simulink model "Simulator_PMU_v4_ons"  (Simulink 8.3)
settings: Solver=FixedStepDiscrete  StartTime=0.0  StopTime=5  FixedStep=1/(60*32)  RelTol=1e-3
undefined symbols (not defined in the file or in its folder): j
libraries: dspbuff3 x5, dspsigops x3, dspxfrm3 x3, simulink x3
settings Model: Creator=dotta  LastModifiedBy=dotta  BufferReuse=off
settings OptimizationCC: BlockReduction=off  InlineParams=on  BufferReuse=off  ExpressionDepthLimit=2147483647
settings DebuggingCC: SigSpecEnsureSampleTimeMsg=none  FcnCallInpInsideContextMsg=UseLocalSettings  StrictBusMsg=Warning
settings SFSimCC: SimParseCustomCode=off

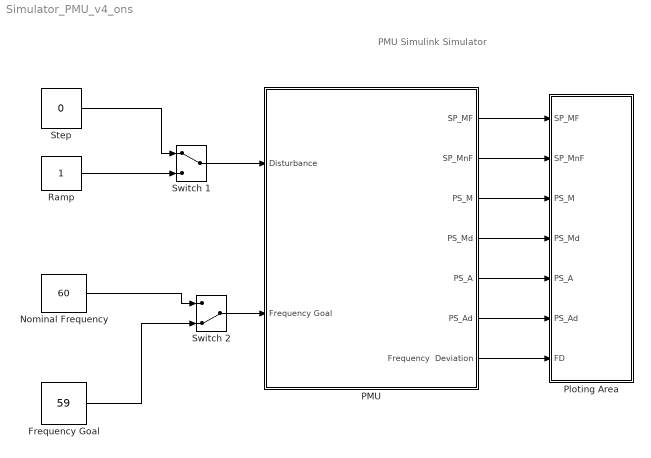
== system Simulator_PMU_v4_ons ==
  note: PMU Simulink Simulator
  Frequency Goal : Constant  Value=59
  Nominal Frequency : Constant  Value=60
  PMU : Subsystem
  Ploting Area : Subsystem
  Ramp : Constant
  Step : Constant  Value=0
  "Switch 1 " : ManualSwitch
  "Switch 2 " : ManualSwitch  CurrentSetting=0
  wires:
  PMU/1(SP_MF) -> Ploting Area/1(SP_MF)
  PMU/2(SP_MnF) -> Ploting Area/2(SP_MnF)
  PMU/4(PS_Md) -> Ploting Area/4(PS_Md)
  PMU/6(PS_Ad) -> Ploting Area/6(PS_Ad)
  Step/1 -> "Switch 1 "/1
  Ramp/1 -> "Switch 1 "/2
  "Switch 2 "/1 -> PMU/2(Frequency Goal)
  PMU/3(PS_M) -> Ploting Area/3(PS_M)
  PMU/5(PS_A) -> Ploting Area/5(PS_A)
  PMU/7(Frequency  Deviation) -> Ploting Area/7(FD)
  Nominal Frequency/1 -> "Switch 2 "/1
  Frequency Goal/1 -> "Switch 2 "/2
  "Switch 1 "/1 -> PMU/1(Disturbance)

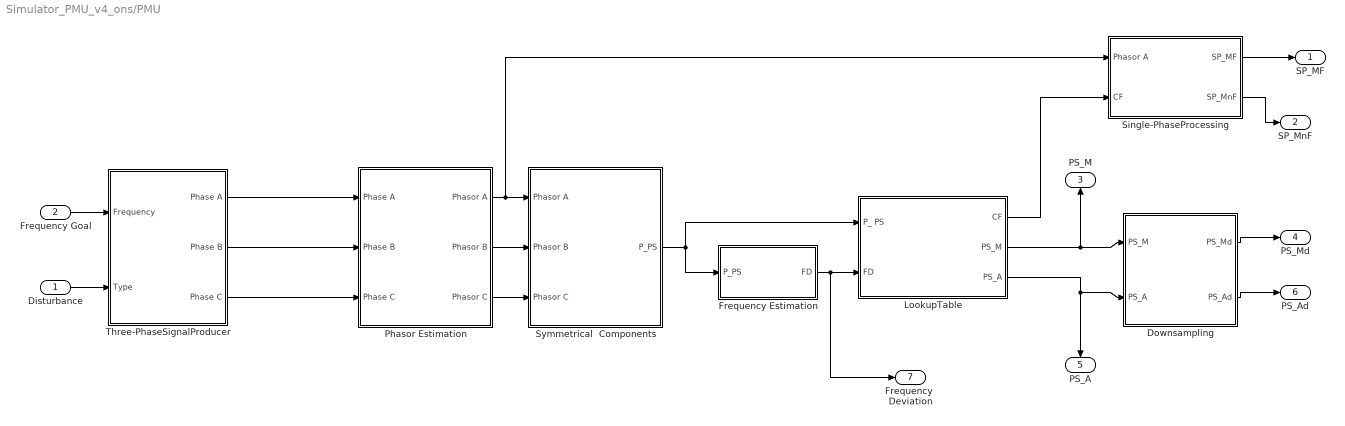
== system Simulator_PMU_v4_ons/PMU ==
  Disturbance : Inport
  Frequency Goal : Inport  Port=2
  Downsampling : Subsystem
  Frequency Estimation : Subsystem
  LookupTable : Subsystem
  Phasor Estimation : Subsystem
  Single-PhaseProcessing : Subsystem
  Symmetrical  Components : Subsystem
  Three-PhaseSignalProducer : Subsystem
  SP_MF : Outport
  SP_MnF : Outport  Port=2
  PS_M : Outport  Port=3
  PS_Md : Outport  Port=4
  PS_A : Outport  Port=5
  PS_Ad : Outport  Port=6
  Frequency  Deviation : Outport  Port=7
  wires:
  Phasor Estimation/1(Phasor A) -> Single-PhaseProcessing/1(Phasor A), Symmetrical  Components/1(Phasor A)
  Symmetrical  Components/1(P_PS) -> Frequency Estimation/1(P_PS), LookupTable/1(P_ PS)
  LookupTable/2(PS_M) -> Downsampling/1(PS_M), PS_M/1
  LookupTable/3(PS_A) -> Downsampling/2(PS_A), PS_A/1
  Frequency Estimation/1(FD) -> LookupTable/2(FD), Frequency  Deviation/1
  LookupTable/1(CF) -> Single-PhaseProcessing/2(CF)
  Phasor Estimation/2(Phasor B) -> Symmetrical  Components/2(Phasor B)
  Phasor Estimation/3(Phasor C) -> Symmetrical  Components/3(Phasor C)
  Single-PhaseProcessing/1(SP_MF) -> SP_MF/1
  Single-PhaseProcessing/2(SP_MnF) -> SP_MnF/1
  Downsampling/1(" PS_Md") -> PS_Md/1
  Frequency Goal/1 -> Three-PhaseSignalProducer/1(Frequency)
  Downsampling/2(PS_Ad) -> PS_Ad/1
  Disturbance/1 -> Three-PhaseSignalProducer/2(Type)
  Three-PhaseSignalProducer/1(Phase A) -> Phasor Estimation/1(" Phase A")
  Three-PhaseSignalProducer/2(Phase B) -> Phasor Estimation/2(Phase B)
  Three-PhaseSignalProducer/3(Phase C) -> Phasor Estimation/3(Phase C)

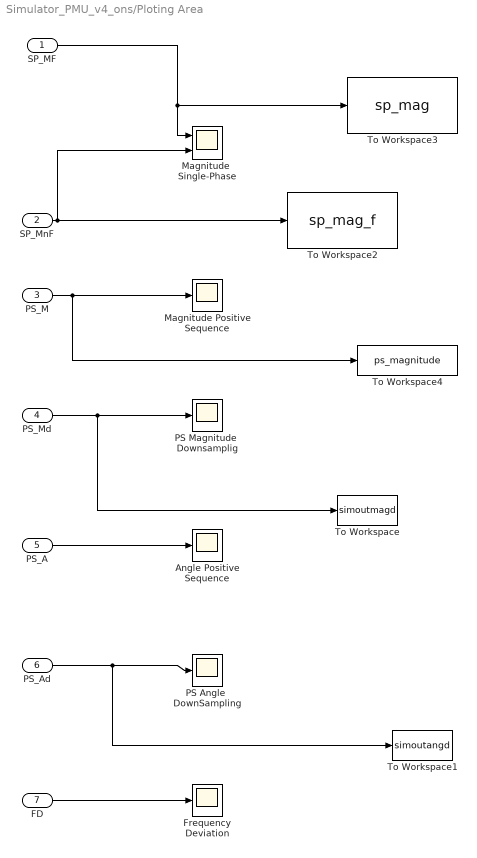
== system Simulator_PMU_v4_ons/Ploting Area ==
  SP_MF : Inport
  SP_MnF : Inport  Port=2
  PS_M : Inport  Port=3
  PS_Md : Inport  Port=4
  PS_A : Inport  Port=5
  PS_Ad : Inport  Port=6
  FD : Inport  Port=7
  Angle Positive Sequence : Scope
      settings: YMin=-3.5  YMax=3.5  SaveName=ScopeData2  MaxDataPoints=10000
  Frequency Deviation : Scope
      settings: YMin=13.85  YMax=15  SaveName=ScopeData3  MaxDataPoints=10000
  Magnitude  Single-Phase : Scope  NumInputPorts=2
      settings: YMin=0.999~0.991  YMax=1.001~1.009  SaveName=ScopeData5  MaxDataPoints=10000
  Magnitude Positive Sequence : Scope
      settings: YMin=0.9993  YMax=1.00025  MaxDataPoints=10000
  PS Angle  DownSampling : Scope
      settings: YMin=-175  YMax=200  SaveName=ScopeData6  MaxDataPoints=10000
  PS Magnitude  Downsamplig : Scope
      settings: YMin=0.95  YMax=1.05  MaxDataPoints=10000
  To Workspace : ToWorkspace  VariableName=simoutmagd  SaveFormat=Structure With Time  SampleTime=-1
  To Workspace1 : ToWorkspace  VariableName=simoutangd  SaveFormat=Structure With Time  SampleTime=-1
  To Workspace2 : ToWorkspace  VariableName=sp_mag_f  SaveFormat=Structure  SampleTime=-1
  To Workspace3 : ToWorkspace  VariableName=sp_mag  SaveFormat=Structure  SampleTime=-1
  To Workspace4 : ToWorkspace  VariableName=ps_magnitude  SaveFormat=Structure With Time  SampleTime=-1
  wires:
  SP_MF/1 -> Magnitude  Single-Phase/1, To Workspace3/1
  SP_MnF/1 -> Magnitude  Single-Phase/2, To Workspace2/1
  PS_M/1 -> Magnitude Positive Sequence/1, To Workspace4/1
  PS_Md/1 -> PS Magnitude  Downsamplig/1, To Workspace/1
  PS_A/1 -> Angle Positive Sequence/1
  PS_Ad/1 -> PS Angle  DownSampling/1, To Workspace1/1
  FD/1 -> Frequency Deviation/1

== system Simulator_PMU_v4_ons/PMU/Downsampling ==
  PS_M : Inport
  PS_A : Inport  Port=2
  Downsample A : dspsigops/Downsample  N=32  phase=0  InputProcessing=Inherited (this choice will be removed - see release notes)  RateOptions=Enforce single-rate processing  smode=Allow multirate  fmode=Maintain input frame size  ic=0
  Downsample M : dspsigops/Downsample  N=32  phase=0  InputProcessing=Inherited (this choice will be removed - see release notes)  RateOptions=Enforce single-rate processing  smode=Allow multirate  fmode=Maintain input frame size  ic=0
  Gain : Gain  Gain=180/pi
  " PS_Md" : Outport
  PS_Ad : Outport  Port=2
  wires:
  Downsample M/1 -> " PS_Md"/1
  PS_M/1 -> Downsample M/1
  PS_A/1 -> Downsample A/1
  Gain/1 -> PS_Ad/1
  Downsample A/1 -> Gain/1

== system Simulator_PMU_v4_ons/PMU/Frequency Estimation ==
  P_PS : Inport
  Complex to Magnitude-Angle : ComplexToMagnitudeAngle  Output=Angle
  Frequency Buffer : dspbuff3/Buffer  N=32*2+1  V=32*2-1  ic=0
  Frequency Datalog : ToWorkspace  VariableName=simoutf  SampleTime=-1
  Frequency  Estimation : MATLABFcn  MATLABFcn=freq_angle  Output1D=off
  FD : Outport
  wires:
  Frequency Buffer/1 -> Frequency  Estimation/1
  Frequency  Estimation/1 -> Frequency Datalog/1, FD/1
  Complex to Magnitude-Angle/1 -> Frequency Buffer/1
  P_PS/1 -> Complex to Magnitude-Angle/1

== system Simulator_PMU_v4_ons/PMU/LookupTable ==
  P_ PS : Inport
  FD : Inport  Port=2
  Complex to Magnitude-Angle : ComplexToMagnitudeAngle
  Divide : Product  Inputs=*/
  P_n Estimation : Subsystem
  Reshape : Reshape
  CF : Outport
  PS_M : Outport  Port=2
  PS_A : Outport  Port=3
  wires:
  Divide/1 -> Complex to Magnitude-Angle/1
  FD/1 -> Reshape/1
  Complex to Magnitude-Angle/1 -> PS_M/1
  Complex to Magnitude-Angle/2 -> PS_A/1
  P_ PS/1 -> Divide/1
  P_n Estimation/1(P_n) -> Divide/2, CF/1
  Reshape/1 -> P_n Estimation/1(Frequency Deviation)

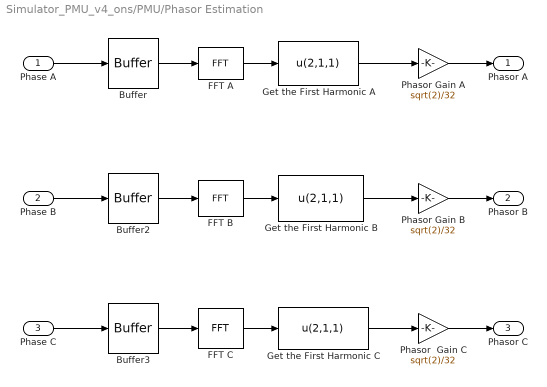
== system Simulator_PMU_v4_ons/PMU/Phasor Estimation ==
  " Phase A" : Inport
  Phase B : Inport  Port=2
  Phase C : Inport  Port=3
  Buffer : dspbuff3/Buffer  N=32  V=31  ic=0
  Buffer2 : dspbuff3/Buffer  N=32  V=31  ic=0
  Buffer3 : dspbuff3/Buffer  N=32  V=31  ic=0
  FFT A : dspxfrm3/FFT  CompMethod=Table lookup  TableOpt=HYBRID  TableOptActive=Speed  BitRevOrder=off  InheritFFTLength=on  FFTLength=31  SkipNorm=off  firstCoeffDataTypeStr=Inherit: Same word length as input  firstCoeffLastDataTypeStr=Inherit: Same word length as input  outputMin=[]  outputMax=[]  roundingMode=Round  overflowMode=off
  FFT B : dspxfrm3/FFT  CompMethod=Table lookup  TableOpt=HYBRID  TableOptActive=Speed  BitRevOrder=off  InheritFFTLength=on  FFTLength=32  SkipNorm=off  firstCoeffDataTypeStr=Inherit: Same word length as input  firstCoeffLastDataTypeStr=Inherit: Same word length as input  outputMin=[]  outputMax=[]  roundingMode=Round  overflowMode=off
  FFT C : dspxfrm3/FFT  CompMethod=Table lookup  TableOpt=HYBRID  TableOptActive=Speed  BitRevOrder=off  InheritFFTLength=on  FFTLength=32  SkipNorm=off  firstCoeffDataTypeStr=Inherit: Same word length as input  firstCoeffLastDataTypeStr=Inherit: Same word length as input  outputMin=[]  outputMax=[]  roundingMode=Round  overflowMode=off
  Get the First Harmonic A : MATLABFcn  MATLABFcn=u(2,1,1)  OutputSignalType=complex
  Get the First Harmonic B : MATLABFcn  MATLABFcn=u(2,1,1)  OutputSignalType=complex
  Get the First Harmonic C : MATLABFcn  MATLABFcn=u(2,1,1)  OutputSignalType=complex
  Phasor Gain A : Gain  Gain=sqrt(2)/32
  Phasor Gain B : Gain  Gain=sqrt(2)/32
  Phasor  Gain C : Gain  Gain=sqrt(2)/32
  Phasor A : Outport
  Phasor B : Outport  Port=2
  Phasor C : Outport  Port=3
  wires:
  FFT A/1 -> Get the First Harmonic A/1
  Buffer/1 -> FFT A/1
  Get the First Harmonic A/1 -> Phasor Gain A/1
  FFT B/1 -> Get the First Harmonic B/1
  Buffer2/1 -> FFT B/1
  Get the First Harmonic B/1 -> Phasor Gain B/1
  FFT C/1 -> Get the First Harmonic C/1
  Buffer3/1 -> FFT C/1
  Get the First Harmonic C/1 -> Phasor  Gain C/1
  " Phase A"/1 -> Buffer/1
  Phasor Gain A/1 -> Phasor A/1
  Phase B/1 -> Buffer2/1
  Phasor Gain B/1 -> Phasor B/1
  Phase C/1 -> Buffer3/1
  Phasor  Gain C/1 -> Phasor C/1

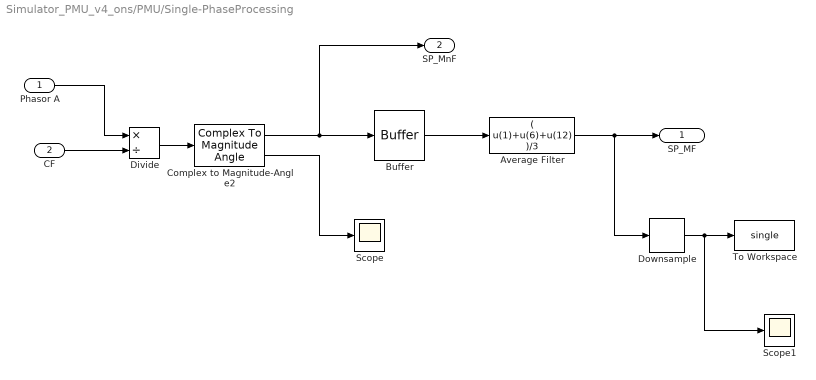
== system Simulator_PMU_v4_ons/PMU/Single-PhaseProcessing ==
  Phasor A : Inport
  CF : Inport  Port=2
  Average Filter : MATLABFcn  MATLABFcn=( u(1)+u(6)+u(12) )/3  Output1D=off
  Buffer : dspbuff3/Buffer  N=32  V=31  ic=0
  Complex to Magnitude-Angle2 : ComplexToMagnitudeAngle
  Divide : Product  Inputs=*/
  Downsample : dspsigops/Downsample  N=32  phase=0  ic=0  smode=Allow multirate  fmode=Maintain input frame size
  Scope : Scope
      settings: SaveName=ScopeData11
  Scope1 : Scope
      settings: SaveName=ScopeData12
  To Workspace : ToWorkspace  VariableName=single  SaveFormat=Structure  SampleTime=-1
  SP_MF : Outport
  SP_MnF : Outport  Port=2
  wires:
  Phasor A/1 -> Divide/1
  CF/1 -> Divide/2
  Complex to Magnitude-Angle2/2 -> Scope/1
  Complex to Magnitude-Angle2/1 -> Buffer/1, SP_MnF/1
  Buffer/1 -> Average Filter/1
  Divide/1 -> Complex to Magnitude-Angle2/1
  Average Filter/1 -> SP_MF/1, Downsample/1
  Downsample/1 -> To Workspace/1, Scope1/1

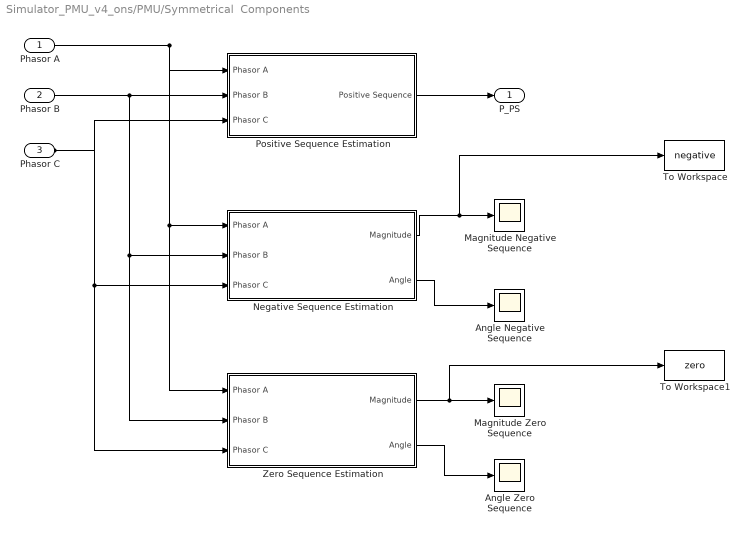
== system Simulator_PMU_v4_ons/PMU/Symmetrical  Components ==
  Phasor A : Inport
  Phasor B : Inport  Port=2
  Phasor C : Inport  Port=3
  Angle Negative Sequence : Scope
      settings: SaveName=ScopeData7
  Angle Zero Sequence : Scope
      settings: SaveName=ScopeData9
  Magnitude Negative Sequence : Scope
      settings: SaveName=ScopeData8  MaxDataPoints=10000
  Magnitude Zero Sequence : Scope
      settings: SaveName=ScopeData10  MaxDataPoints=10000
  Negative Sequence Estimation : Subsystem
  Positive Sequence Estimation : Subsystem
  To Workspace : ToWorkspace  VariableName=negative  SaveFormat=Structure  SampleTime=-1
  To Workspace1 : ToWorkspace  VariableName=zero  SaveFormat=Structure  SampleTime=-1
  Zero Sequence Estimation : Subsystem
  P_PS : Outport
  wires:
  Phasor C/1 -> Zero Sequence Estimation/3(Phasor C), Negative Sequence Estimation/3(Phasor C), Positive Sequence Estimation/3(Phasor C)
  Phasor B/1 -> Zero Sequence Estimation/2(Phasor B), Negative Sequence Estimation/2(Phasor B), Positive Sequence Estimation/2(Phasor B)
  Negative Sequence Estimation/2(Angle) -> Angle Negative Sequence/1
  Negative Sequence Estimation/1(Magnitude) -> Magnitude Negative Sequence/1, To Workspace/1
  Zero Sequence Estimation/2(Angle) -> Angle Zero Sequence/1
  Zero Sequence Estimation/1(Magnitude) -> Magnitude Zero Sequence/1, To Workspace1/1
  Phasor A/1 -> Positive Sequence Estimation/1(Phasor A), Negative Sequence Estimation/1(Phasor A), Zero Sequence Estimation/1(Phasor A)
  Positive Sequence Estimation/1(Positive Sequence) -> P_PS/1

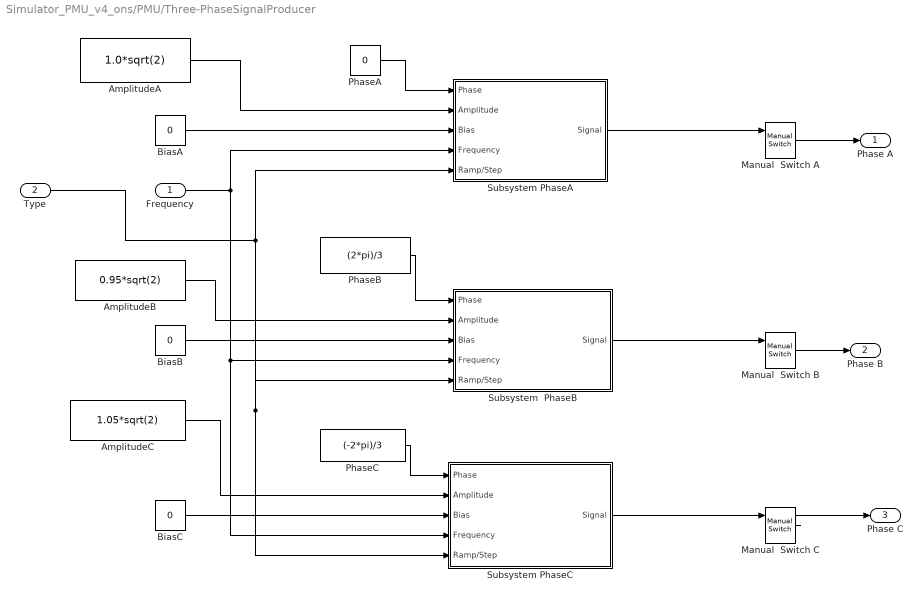
== system Simulator_PMU_v4_ons/PMU/Three-PhaseSignalProducer ==
  Frequency : Inport
  Type : Inport  Port=2
  AmplitudeA : Constant  Value=1.0*sqrt(2)
  AmplitudeB : Constant  Value=0.95*sqrt(2)
  AmplitudeC : Constant  Value=1.05*sqrt(2)
  BiasA : Constant  Value=0
  BiasB : Constant  Value=0
  BiasC : Constant  Value=0
  Manual  Switch A : simulink/Signal Routing/Manual Switch  SystemSampleTime=-1  sw=1  action=0  varsize=off
  Manual  Switch B : simulink/Signal Routing/Manual Switch  SystemSampleTime=-1  sw=1  action=0  varsize=off
  Manual  Switch C : simulink/Signal Routing/Manual Switch  SystemSampleTime=-1  sw=1  action=0  varsize=off
  PhaseA : Constant  Value=0
  PhaseB : Constant  Value=(2*pi)/3
  PhaseC : Constant  Value=(-2*pi)/3
  Subsystem PhaseA : Subsystem
  Subsystem PhaseC : Subsystem
  Subsystem  PhaseB : Subsystem
  Phase A : Outport
  Phase B : Outport  Port=2
  Phase C : Outport  Port=3
  wires:
  AmplitudeB/1 -> Subsystem  PhaseB/2(Amplitude)
  BiasB/1 -> Subsystem  PhaseB/3(Bias)
  PhaseB/1 -> Subsystem  PhaseB/1(Phase)
  AmplitudeC/1 -> Subsystem PhaseC/2(Amplitude)
  BiasC/1 -> Subsystem PhaseC/3(Bias)
  PhaseC/1 -> Subsystem PhaseC/1(Phase)
  BiasA/1 -> Subsystem PhaseA/3(Bias)
  PhaseA/1 -> Subsystem PhaseA/1(Phase)
  AmplitudeA/1 -> Subsystem PhaseA/2(Amplitude)
  Frequency/1 -> Subsystem PhaseA/4(Frequency), Subsystem  PhaseB/4(Frequency), Subsystem PhaseC/4(Frequency)
  Type/1 -> Subsystem PhaseA/5(Ramp/Step), Subsystem  PhaseB/5(Ramp/Step), Subsystem PhaseC/5(Ramp/Step)
  Subsystem PhaseC/1(Signal) -> Manual  Switch C/1
  Manual  Switch C/1 -> Phase C/1
  Manual  Switch B/1 -> Phase B/1
  Subsystem  PhaseB/1(Signal) -> Manual  Switch B/1
  Manual  Switch A/1 -> Phase A/1
  Subsystem PhaseA/1("Signal ") -> Manual  Switch A/1

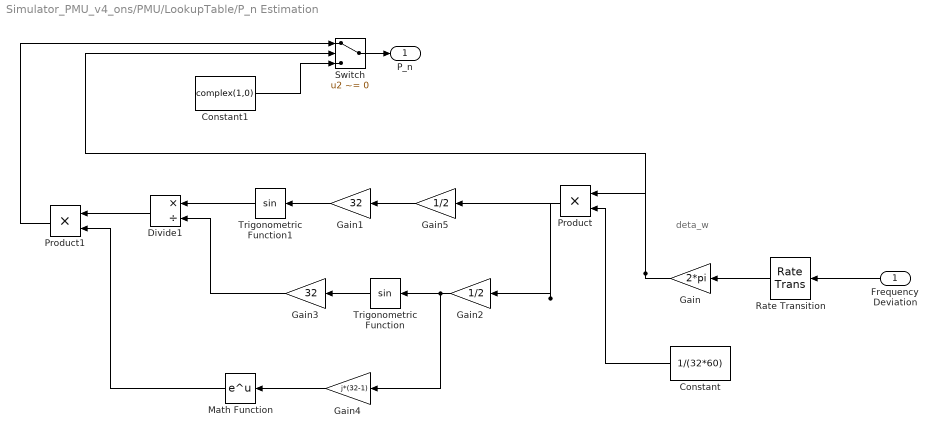
== system Simulator_PMU_v4_ons/PMU/LookupTable/P_n Estimation ==
  note: deta_w
  Frequency Deviation : Inport
  Constant : Constant  Value=1/(32*60)
  Constant1 : Constant  Value=complex(1,0)  VectorParams1D=off
  Divide1 : Product  Inputs=*/
  Gain : Gain  Gain=2*pi  SampleTime=1/(32*60)
  Gain1 : Gain  Gain=32
  Gain2 : Gain  Gain=1/2
  Gain3 : Gain  Gain=32
  Gain4 : Gain  Gain=j*(32-1)
  Gain5 : Gain  Gain=1/2
  Math Function : Math  SaturateOnIntegerOverflow=on
  Product : Product  RndMeth=Zero
  Product1 : Product  RndMeth=Zero
  Rate Transition : RateTransition  OutPortSampleTime=1/(32*60)
  Switch : Switch  Criteria=u2 ~= 0
  Trigonometric Function : Trigonometry
  Trigonometric Function1 : Trigonometry
  P_n : Outport
  wires:
  Gain/1 -> Product/1, Switch/2
  Constant/1 -> Product/2
  Product/1 -> Gain2/1, Gain5/1
  Gain2/1 -> Trigonometric Function/1, Gain4/1
  Trigonometric Function/1 -> Gain3/1
  Gain1/1 -> Trigonometric Function1/1
  Gain3/1 -> Divide1/2
  Trigonometric Function1/1 -> Divide1/1
  Gain4/1 -> Math Function/1
  Product1/1 -> Switch/1
  Constant1/1 -> Switch/3
  Gain5/1 -> Gain1/1
  Rate Transition/1 -> Gain/1
  Divide1/1 -> Product1/1
  Math Function/1 -> Product1/2
  Switch/1 -> P_n/1
  Frequency Deviation/1 -> Rate Transition/1

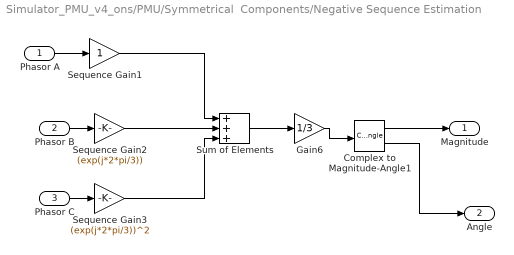
== system Simulator_PMU_v4_ons/PMU/Symmetrical  Components/Negative Sequence Estimation ==
  Phasor A : Inport
  Phasor B : Inport  Port=2
  Phasor C : Inport  Port=3
  Complex to Magnitude-Angle1 : ComplexToMagnitudeAngle
  Gain6 : Gain  Gain=1/3  SampleTime=1/(32*60)
  Sequence Gain1 : Gain
  Sequence Gain2 : Gain  Gain=(exp(j*2*pi/3))
  Sequence Gain3 : Gain  Gain=(exp(j*2*pi/3))^2
  Sum of Elements : Sum  Inputs=+++
  Magnitude : Outport
  Angle : Outport  Port=2
  wires:
  Sequence Gain1/1 -> Sum of Elements/1
  Sequence Gain2/1 -> Sum of Elements/2
  Sequence Gain3/1 -> Sum of Elements/3
  Sum of Elements/1 -> Gain6/1
  Phasor A/1 -> Sequence Gain1/1
  Gain6/1 -> Complex to Magnitude-Angle1/1
  Phasor B/1 -> Sequence Gain2/1
  Phasor C/1 -> Sequence Gain3/1
  Complex to Magnitude-Angle1/1 -> Magnitude/1
  Complex to Magnitude-Angle1/2 -> Angle/1

== system Simulator_PMU_v4_ons/PMU/Symmetrical  Components/Positive Sequence Estimation ==
  Phasor A : Inport
  Phasor B : Inport  Port=2
  Phasor C : Inport  Port=3
  Gain6 : Gain  Gain=1/3  SampleTime=1/(32*60)
  Sequence Gain1 : Gain
  Sequence Gain2 : Gain  Gain=(exp(j*2*pi/3))^2
  Sequence Gain3 : Gain  Gain=exp(j*2*pi/3)
  Sum of Elements : Sum  Inputs=+++
  Positive Sequence : Outport
  wires:
  Sequence Gain1/1 -> Sum of Elements/1
  Sequence Gain2/1 -> Sum of Elements/2
  Sequence Gain3/1 -> Sum of Elements/3
  Sum of Elements/1 -> Gain6/1
  Phasor A/1 -> Sequence Gain1/1
  Gain6/1 -> Positive Sequence/1
  Phasor B/1 -> Sequence Gain2/1
  Phasor C/1 -> Sequence Gain3/1

== system Simulator_PMU_v4_ons/PMU/Symmetrical  Components/Zero Sequence Estimation ==
  Phasor A : Inport
  Phasor B : Inport  Port=2
  Phasor C : Inport  Port=3
  Complex to Magnitude-Angle1 : ComplexToMagnitudeAngle
  Gain6 : Gain  Gain=1/3  SampleTime=1/(32*60)
  Sequence Gain1 : Gain
  Sequence Gain2 : Gain
  Sequence Gain3 : Gain
  Sum of Elements : Sum  Inputs=+++
  Magnitude : Outport
  Angle : Outport  Port=2
  wires:
  Sequence Gain1/1 -> Sum of Elements/1
  Sequence Gain2/1 -> Sum of Elements/2
  Sequence Gain3/1 -> Sum of Elements/3
  Sum of Elements/1 -> Gain6/1
  Phasor A/1 -> Sequence Gain1/1
  Gain6/1 -> Complex to Magnitude-Angle1/1
  Phasor B/1 -> Sequence Gain2/1
  Phasor C/1 -> Sequence Gain3/1
  Complex to Magnitude-Angle1/1 -> Magnitude/1
  Complex to Magnitude-Angle1/2 -> Angle/1

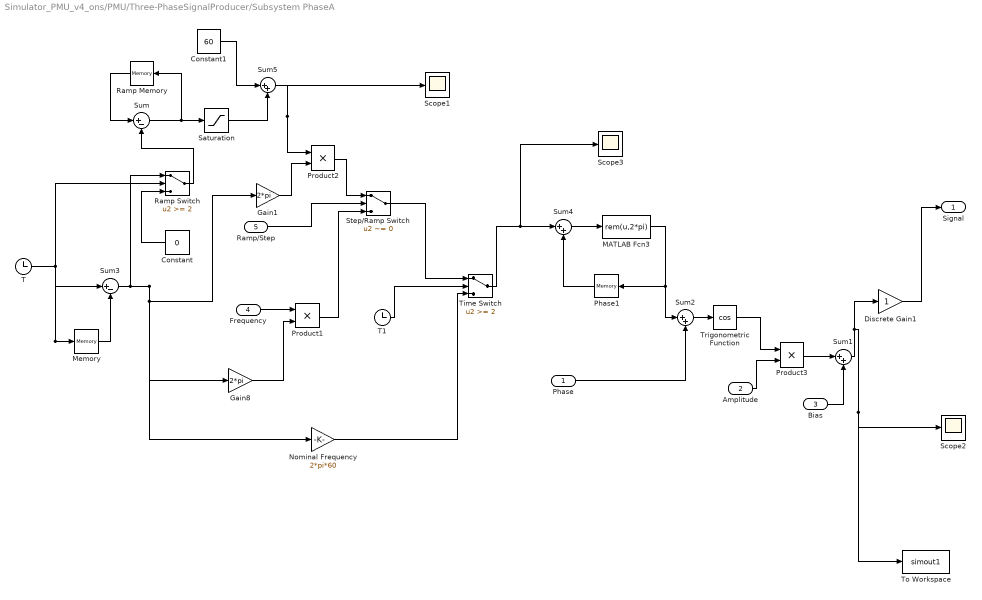
== system Simulator_PMU_v4_ons/PMU/Three-PhaseSignalProducer/Subsystem PhaseA ==
  Phase : Inport
  Amplitude : Inport  Port=2
  Bias : Inport  Port=3
  Frequency : Inport  Port=4
  Ramp/Step : Inport  Port=5
  Constant : Constant  Value=0
  Constant1 : Constant  Value=60
  Discrete Gain1 : Gain  SampleTime=1/(32*60)
  Gain1 : Gain  Gain=2*pi
  Gain8 : Gain  Gain=2*pi
  MATLAB Fcn3 : MATLABFcn  MATLABFcn=rem(u,2*pi)
  Memory : Memory
  Nominal Frequency : Gain  Gain=2*pi*60
  Phase1 : Memory  X0=-(2*pi)/32  LinearizeMemory=on
  Product1 : Product  RndMeth=Zero
  Product2 : Product  RndMeth=Zero
  Product3 : Product  RndMeth=Zero
  Ramp Memory : Memory
  Ramp Switch : Switch  Threshold=2
  Saturation : Saturate  UpperLimit=1  LowerLimit=-1
  Scope1 : Scope
      settings: SaveName=ScopeData4  MaxDataPoints=10000
  Scope2 : Scope
      settings: YMin=-1.5  YMax=1.5  SaveName=ScopeData14  MaxDataPoints=10000
  Scope3 : Scope
      settings: SaveName=ScopeData15  MaxDataPoints=10000
  Step/Ramp Switch : Switch  Criteria=u2 ~= 0  Threshold=2
  Sum : Sum  Inputs=|+-
  Sum{1..2,4..5} (4 alike) : Sum  Inputs=|++
  Sum3 : Sum  Inputs=|+-
  T : Clock
  T1 : Clock
  Time Switch : Switch  Threshold=2
  To Workspace : ToWorkspace  VariableName=simout1  SaveFormat=Structure  SampleTime=-1
  Trigonometric Function : Trigonometry  Operator=cos
  "Signal " : Outport
  wires:
  Trigonometric Function/1 -> Product3/1
  Product3/1 -> Sum1/1
  T/1 -> Memory/1, Sum3/1, Ramp Switch/2
  Sum3/1 -> Ramp Switch/1, Nominal Frequency/1, Gain8/1, Gain1/1
  Phase1/1 -> Sum4/2
  Sum4/1 -> MATLAB Fcn3/1
  MATLAB Fcn3/1 -> Phase1/1, Sum2/1
  Nominal Frequency/1 -> Time Switch/3
  Time Switch/1 -> Sum4/1, Scope3/1
  Sum/1 -> Ramp Memory/1, Saturation/1
  Ramp Memory/1 -> Sum/1
  Ramp Switch/1 -> Sum/2
  Constant/1 -> Ramp Switch/3
  Product2/1 -> Step/Ramp Switch/1
  Step/Ramp Switch/1 -> Time Switch/1
  T1/1 -> Time Switch/2
  Memory/1 -> Sum3/2
  Sum2/1 -> Trigonometric Function/1
  Phase/1 -> Sum2/2
  Amplitude/1 -> Product3/2
  Bias/1 -> Sum1/2
  Discrete Gain1/1 -> "Signal "/1
  Sum1/1 -> Discrete Gain1/1, Scope2/1, To Workspace/1
  Gain8/1 -> Product1/2
  Product1/1 -> Step/Ramp Switch/3
  Frequency/1 -> Product1/1
  Ramp/Step/1 -> Step/Ramp Switch/2
  Sum5/1 -> Product2/1, Scope1/1
  Saturation/1 -> Sum5/2
  Constant1/1 -> Sum5/1
  Gain1/1 -> Product2/2

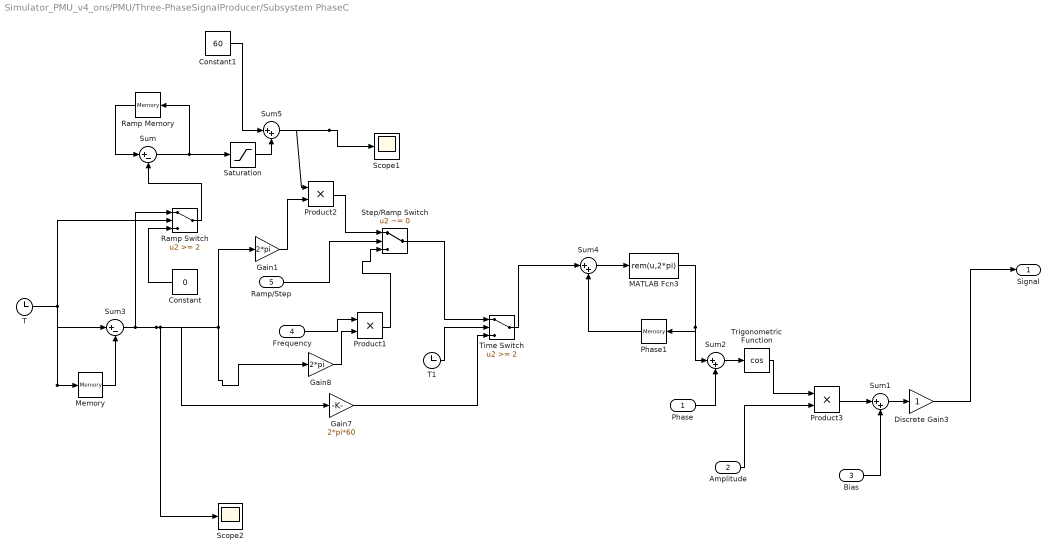
== system Simulator_PMU_v4_ons/PMU/Three-PhaseSignalProducer/Subsystem PhaseC ==
  Phase : Inport
  Amplitude : Inport  Port=2
  Bias : Inport  Port=3
  Frequency : Inport  Port=4
  Ramp/Step : Inport  Port=5
  Constant : Constant  Value=0
  Constant1 : Constant  Value=60
  Discrete Gain3 : Gain  SampleTime=1/(32*60)
  Gain1 : Gain  Gain=2*pi
  Gain7 : Gain  Gain=2*pi*60
  Gain8 : Gain  Gain=2*pi
  MATLAB Fcn3 : MATLABFcn  MATLABFcn=rem(u,2*pi)
  Memory : Memory
  Phase1 : Memory  X0=-(2*pi)/32
  Product1 : Product  RndMeth=Zero
  Product2 : Product  RndMeth=Zero
  Product3 : Product  RndMeth=Zero
  Ramp Memory : Memory
  Ramp Switch : Switch  Threshold=2
  Saturation : Saturate  UpperLimit=1  LowerLimit=-1
  Scope1 : Scope
      settings: SaveName=ScopeData4
  Scope2 : Scope
      settings: YMin=-2.71051e-020  YMax=0.000525  SaveName=ScopeData13
  Step/Ramp Switch : Switch  Criteria=u2 ~= 0  Threshold=2
  Sum : Sum  Inputs=|+-
  Sum{1..2,4..5} (4 alike) : Sum  Inputs=|++
  Sum3 : Sum  Inputs=|+-
  T : Clock
  T1 : Clock
  Time Switch : Switch  Threshold=2
  Trigonometric Function : Trigonometry  Operator=cos
  Signal : Outport
  wires:
  Trigonometric Function/1 -> Product3/1
  Product3/1 -> Sum1/1
  T/1 -> Memory/1, Sum3/1, Ramp Switch/2
  Sum3/1 -> Ramp Switch/1, Gain7/1, Gain8/1, Gain1/1, Scope2/1
  Phase1/1 -> Sum4/2
  Sum4/1 -> MATLAB Fcn3/1
  MATLAB Fcn3/1 -> Phase1/1, Sum2/1
  Gain7/1 -> Time Switch/3
  Time Switch/1 -> Sum4/1
  Sum/1 -> Ramp Memory/1, Saturation/1
  Ramp Memory/1 -> Sum/1
  Ramp Switch/1 -> Sum/2
  Constant/1 -> Ramp Switch/3
  Product2/1 -> Step/Ramp Switch/1
  Step/Ramp Switch/1 -> Time Switch/1
  T1/1 -> Time Switch/2
  Memory/1 -> Sum3/2
  Sum2/1 -> Trigonometric Function/1
  Phase/1 -> Sum2/2
  Amplitude/1 -> Product3/2
  Bias/1 -> Sum1/2
  Sum1/1 -> Discrete Gain3/1
  Discrete Gain3/1 -> Signal/1
  Product1/1 -> Step/Ramp Switch/3
  Frequency/1 -> Product1/1
  Gain8/1 -> Product1/2
  Ramp/Step/1 -> Step/Ramp Switch/2
  Saturation/1 -> Sum5/2
  Sum5/1 -> Scope1/1, Product2/1
  Constant1/1 -> Sum5/1
  Gain1/1 -> Product2/2

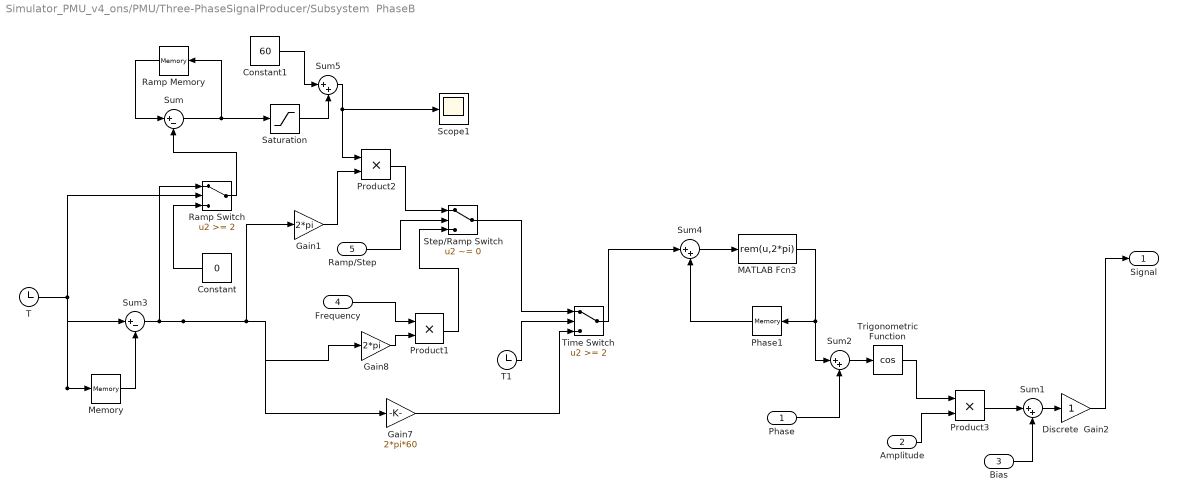
== system Simulator_PMU_v4_ons/PMU/Three-PhaseSignalProducer/Subsystem  PhaseB ==
  Phase : Inport
  Amplitude : Inport  Port=2
  Bias : Inport  Port=3
  Frequency : Inport  Port=4
  Ramp/Step : Inport  Port=5
  Constant : Constant  Value=0
  Constant1 : Constant  Value=60
  Discrete  Gain2 : Gain  SampleTime=1/(32*60)
  Gain1 : Gain  Gain=2*pi
  Gain7 : Gain  Gain=2*pi*60
  Gain8 : Gain  Gain=2*pi
  MATLAB Fcn3 : MATLABFcn  MATLABFcn=rem(u,2*pi)
  Memory : Memory
  Phase1 : Memory  X0=-(2*pi)/32
  Product1 : Product  RndMeth=Zero
  Product2 : Product  RndMeth=Zero
  Product3 : Product  RndMeth=Zero
  Ramp Memory : Memory
  Ramp Switch : Switch  Threshold=2
  Saturation : Saturate  UpperLimit=1  LowerLimit=-1
  Scope1 : Scope
      settings: YMin=61  YMax=61  SaveName=ScopeData4  MaxDataPoints=10000
  Step/Ramp Switch : Switch  Criteria=u2 ~= 0  Threshold=2
  Sum : Sum  Inputs=|+-
  Sum{1..2,4..5} (4 alike) : Sum  Inputs=|++
  Sum3 : Sum  Inputs=|+-
  T : Clock
  T1 : Clock
  Time Switch : Switch  Threshold=2
  Trigonometric Function : Trigonometry  Operator=cos
  Signal : Outport
  wires:
  Trigonometric Function/1 -> Product3/1
  Product3/1 -> Sum1/1
  T/1 -> Memory/1, Sum3/1, Ramp Switch/2
  Sum3/1 -> Ramp Switch/1, Gain7/1, Gain8/1, Gain1/1
  Phase1/1 -> Sum4/2
  Sum4/1 -> MATLAB Fcn3/1
  MATLAB Fcn3/1 -> Phase1/1, Sum2/1
  Gain7/1 -> Time Switch/3
  Time Switch/1 -> Sum4/1
  Sum/1 -> Ramp Memory/1, Saturation/1
  Ramp Memory/1 -> Sum/1
  Ramp Switch/1 -> Sum/2
  Constant/1 -> Ramp Switch/3
  Product2/1 -> Step/Ramp Switch/1
  Step/Ramp Switch/1 -> Time Switch/1
  T1/1 -> Time Switch/2
  Memory/1 -> Sum3/2
  Sum2/1 -> Trigonometric Function/1
  Phase/1 -> Sum2/2
  Amplitude/1 -> Product3/2
  Bias/1 -> Sum1/2
  Discrete  Gain2/1 -> Signal/1
  Sum1/1 -> Discrete  Gain2/1
  Product1/1 -> Step/Ramp Switch/3
  Frequency/1 -> Product1/1
  Gain8/1 -> Product1/2
  Ramp/Step/1 -> Step/Ramp Switch/2
  Saturation/1 -> Sum5/2
  Sum5/1 -> Product2/1, Scope1/1
  Constant1/1 -> Sum5/1
  Gain1/1 -> Product2/2
